simulink model "TwoSpeedShiftControllers"  (Simulink 8.6)
settings: Solver=ode45  StartTime=0.0  StopTime=10.0  RelTol=1e-3
settings Model: Creator=choff  LastModifiedBy=CraigAdmin
settings DataIOCC: SignalLoggingSaveFormat=Dataset
settings OptimizationCC: ExpressionDepthLimit=128
settings DebuggingCC: FcnCallInpInsideContextMsg=EnableAllAsError  StateNameClashWarn=none
settings GRTTargetCC: CombineOutputUpdateFcns=on  GRTInterface=off

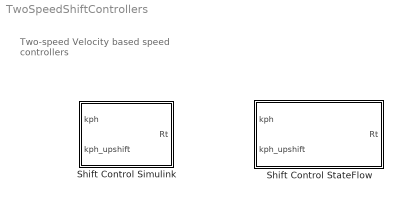
== system TwoSpeedShiftControllers ==
  note: Two-speed
      | Velocity based speed controllers
  Shift Control Simulink : Subsystem
  Shift Control StateFlow : Stateflow chart  TreatAsAtomicUnit=on

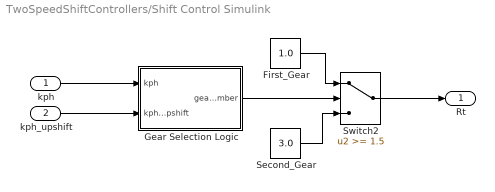
== system TwoSpeedShiftControllers/Shift Control Simulink ==
  kph : Inport
  kph_upshift : Inport  Port=2
  First_Gear : Constant  Value=1.0
  Gear Selection Logic : Subsystem
  Second_Gear : Constant  Value=3.0
  Switch2 : Switch  Threshold=1.5  SaturateOnIntegerOverflow=on  InputSameDT=on
  Rt : Outport
  wires:
  First_Gear/1 -> Switch2/1
  Second_Gear/1 -> Switch2/3
  Switch2/1 -> Rt/1
  kph/1 -> Gear Selection Logic/1(kph)
  kph_upshift/1 -> Gear Selection Logic/2(kph_upshift)
  Gear Selection Logic/1(gear number) -> Switch2/2

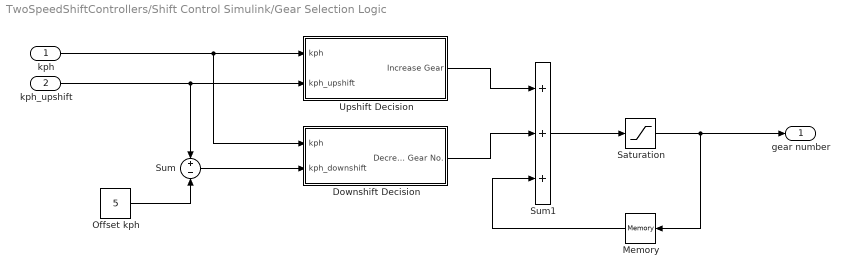
== system TwoSpeedShiftControllers/Shift Control Simulink/Gear Selection Logic ==
  kph : Inport
  kph_upshift : Inport  Port=2
  Downshift Decision : Subsystem
  Memory : Memory
  Offset kph : Constant  Value=5
  Saturation : Saturate  UpperLimit=2  LowerLimit=1
  Sum : Sum  Inputs=+|-
  Sum1 : Sum  Inputs=+++  SaturateOnIntegerOverflow=on  InputSameDT=on  OutDataTypeStr=Inherit: Same as first input
  Upshift Decision : Subsystem
  gear number : Outport
  wires:
  kph_upshift/1 -> Sum/1, Upshift Decision/2(kph_upshift)
  Offset kph/1 -> Sum/2
  Saturation/1 -> gear number/1, Memory/1
  Memory/1 -> Sum1/3
  Sum1/1 -> Saturation/1
  kph/1 -> Downshift Decision/1(kph), Upshift Decision/1(kph)
  Sum/1 -> Downshift Decision/2(kph_downshift)
  Downshift Decision/1(Decrease  Gear No.) -> Sum1/2
  Upshift Decision/1(Increase Gear) -> Sum1/1

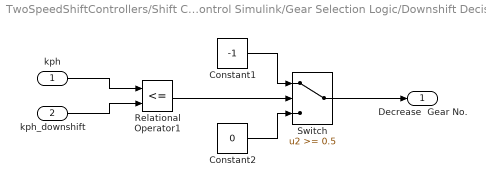
== system TwoSpeedShiftControllers/Shift Control Simulink/Gear Selection Logic/Downshift Decision ==
  kph : Inport
  kph_downshift : Inport  Port=2
  Constant1 : Constant  Value=-1
  Constant2 : Constant  Value=0
  Relational Operator1 : RelationalOperator  Operator=<=  OutDataTypeStr=boolean
  Switch : Switch  Threshold=0.5  SaturateOnIntegerOverflow=on  InputSameDT=on
  Decrease  Gear No. : Outport
  wires:
  Constant2/1 -> Switch/3
  kph_downshift/1 -> Relational Operator1/2
  Constant1/1 -> Switch/1
  Relational Operator1/1 -> Switch/2
  Switch/1 -> Decrease  Gear No./1
  kph/1 -> Relational Operator1/1

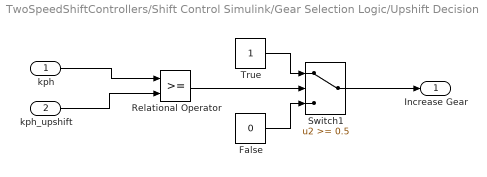
== system TwoSpeedShiftControllers/Shift Control Simulink/Gear Selection Logic/Upshift Decision ==
  kph : Inport
  kph_upshift : Inport  Port=2
  False : Constant  Value=0
  Relational Operator : RelationalOperator  OutDataTypeStr=boolean
  Switch1 : Switch  Threshold=0.5  SaturateOnIntegerOverflow=on  InputSameDT=on
  True : Constant
  Increase Gear : Outport
  wires:
  False/1 -> Switch1/3
  True/1 -> Switch1/1
  Relational Operator/1 -> Switch1/2
  Switch1/1 -> Increase Gear/1
  kph_upshift/1 -> Relational Operator/2
  kph/1 -> Relational Operator/1

== stateflow chart Shift Control StateFlow ==
  state first_gear
    entry: Rt = 3.0;
  state second_gear
    entry: Rt = 1.0;
  (default) -> first_gear
  first_gear -> second_gear : [kph>kph_upshift]
  second_gear -> first_gear : [kph<kph_upshift-5]
  data: kph input double; Rt output double; kph_upshift input double
